simulink model "EOM"  (R2020a)
settings: Solver=VariableStepAuto  StartTime=0.0  StopTime=10.0  RelTol=1e-3
undefined symbols (not defined in the file): itki, Iyy, pos_ini, theta_ini, velbody_ini
libraries: simulink x1, aerolibatmos2 x1
settings Model: Creator=Emir  LastModifiedBy=benyo
settings DebuggingCC: UnconnectedInputMsg=none  UnconnectedOutputMsg=none  UnconnectedLineMsg=none  SFMachineParentedDataDiag=error

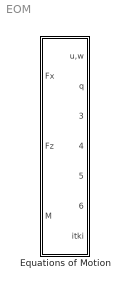
== system EOM ==
  Equations of Motion : Subsystem

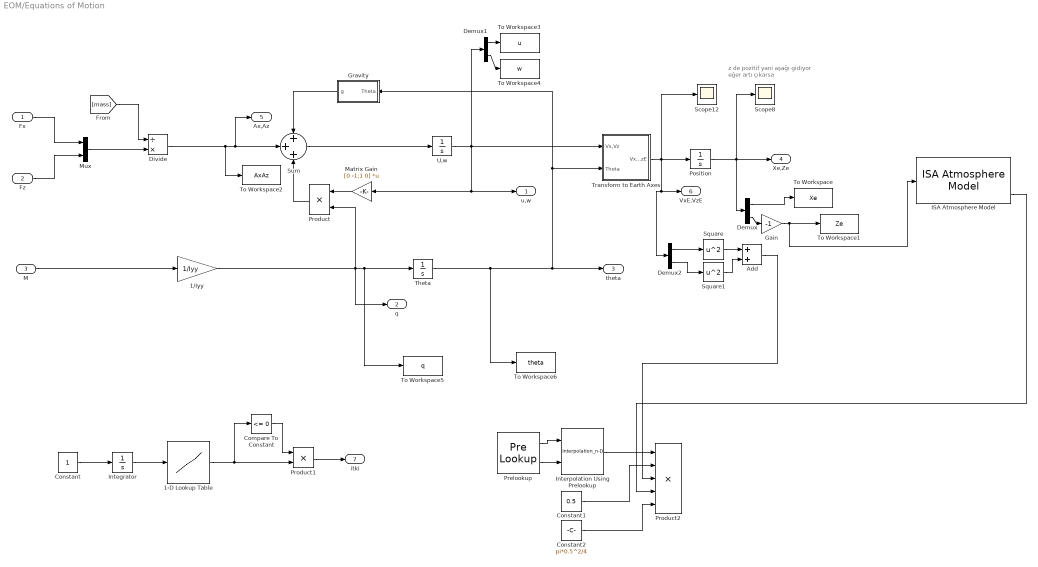
== system EOM/Equations of Motion ==
  note: z de pozitif yani aşağı
      | gidiyor eğer artı çıkarsa
  Fx : Inport
  Fz : Inport  Port=2
  M : Inport  Port=3
  1-D Lookup Table : Lookup_n-D  NumberOfTableDimensions=1  BreakpointsForDimension1=t  Table=itki  InternalRulePriority=Speed  RndMeth=Simplest  InputSameDT=on
  1/Iyy : Gain  Gain=1/Iyy  SaturateOnIntegerOverflow=on  OutDataTypeStr=Inherit: Same as input  ParamDataTypeStr=Inherit: Same as input
  Add : Sum
  Compare To Constant : simulink/Logic and Bit Operations/Compare To Constant  relop=<=  const=0  OutDataTypeStr=boolean
  Constant : Constant
  Constant1 : Constant  Value=0.5
  Constant2 : Constant  Value=pi*0.5^2/4
  Demux : Demux  Outputs=2
  Demux1 : Demux  Outputs=2
  Demux2 : Demux  Outputs=2
  Divide : Product  Inputs=/*
  Gain : Gain  Gain=-1
  Gravity : Subsystem
  ISA Atmosphere Model : aerolibatmos2/ISA Atmosphere Model  custom=off  g=9.80665  gamma=1.4  R=287.0531  L=0.0065  h_trop=11000  h_strat=20000  rho0=1.225  P0=101325  T0=288.15  h0=0
  Integrator : Integrator
  Interpolation Using Prelookup : Interpolation_n-D  NumberOfTableDimensions=1  InternalRulePriority=Speed
      settings: InputPortMap=u0,u1
  Matrix Gain : Gain  Gain=[0 -1;1 0]  Multiplication=Matrix(K*u)  SaturateOnIntegerOverflow=on  OutDataTypeStr=Inherit: Same as input  ParamDataTypeStr=Inherit: Same as input
  Mux : Mux  Inputs=2
  Position : Integrator  InitialCondition=pos_ini
  Prelookup : PreLookup  BreakpointsData=[10:10:110]  ExtrapMethod=Linear
  Product : Product  InputSameDT=on  RndMeth=Zero  SaturateOnIntegerOverflow=on  OutDataTypeStr=Inherit: Same as first input
  Product1 : Product
  Product2 : Product  Inputs=5
  Scope12 : Scope
  Scope8 : Scope
  Square : Math  Operator=square  SaturateOnIntegerOverflow=on
  Square1 : Math  Operator=square  SaturateOnIntegerOverflow=on
  Sum : Sum  Inputs=+++  InputSameDT=on  SaturateOnIntegerOverflow=on  OutDataTypeStr=Inherit: Same as first input
  Theta : Integrator  InitialCondition=theta_ini
  To Workspace : ToWorkspace  VariableName=Xe  SampleTime=-1
  To Workspace1 : ToWorkspace  VariableName=Ze  SampleTime=-1
  To Workspace2 : ToWorkspace  VariableName=AxAz  SaveFormat=Timeseries  SampleTime=-1
  To Workspace3 : ToWorkspace  VariableName=u  SaveFormat=Timeseries  SampleTime=-1
  To Workspace4 : ToWorkspace  VariableName=w  SaveFormat=Timeseries  SampleTime=-1
  To Workspace5 : ToWorkspace  VariableName=q  SampleTime=-1
  To Workspace6 : ToWorkspace  VariableName=theta  SampleTime=-1
  Transform to Earth Axes : Subsystem
  U,w : Integrator  InitialCondition=velbody_ini
  u,w : Outport
  q : Outport  Port=2
  theta : Outport  Port=3
  Xe,Ze : Outport  Port=4  InitialOutput=0
  Ax,Az : Outport  Port=5
  VxE,VzE : Outport  Port=6  InitialOutput=0
  itki : Outport  Port=7
  wires:
  Fx/1 -> Mux/1
  Fz/1 -> Mux/2
  Mux/1 -> Divide/2
  Divide/1 -> Sum/2, Ax,Az/1, To Workspace2/1
  Product/1 -> Sum/3
  Matrix Gain/1 -> Product/1
  1/Iyy/1 -> q/1, Theta/1, To Workspace5/1, Product/2
  Sum/1 -> U,w/1
  Theta/1 -> theta/1, Gravity/1(Theta), Transform to Earth Axes/2(Theta), To Workspace6/1
  Gravity/1(g) -> Sum/1
  U,w/1 -> Transform to Earth Axes/1(Vx,Vz), Matrix Gain/1, u,w/1, Demux1/1
  M/1 -> 1/Iyy/1
  Position/1 -> Scope8/1, Xe,Ze/1, Demux/1
  Transform to Earth Axes/1(VxE,VzE) -> Position/1, Scope12/1, VxE,VzE/1, Demux2/1
  [mass] -> Divide/1
  Demux/1 -> To Workspace/1
  Demux/2 -> Gain/1
  Gain/1 -> To Workspace1/1, ISA Atmosphere Model/1
  Demux1/1 -> To Workspace3/1
  Demux1/2 -> To Workspace4/1
  Constant/1 -> Integrator/1
  Integrator/1 -> 1-D Lookup Table/1
  1-D Lookup Table/1 -> Compare To Constant/1, Product1/2
  Compare To Constant/1 -> Product1/1
  Product1/1 -> itki/1
  Prelookup/1 -> Interpolation Using Prelookup/1
  Prelookup/2 -> Interpolation Using Prelookup/2
  Interpolation Using Prelookup/1 -> Product2/1
  Constant1/1 -> Product2/2
  Demux2/1 -> Square/1
  Demux2/2 -> Square1/1
  Square/1 -> Add/1
  Square1/1 -> Add/2
  Add/1 -> Product2/3
  ISA Atmosphere Model/4 -> Product2/4
  Constant2/1 -> Product2/5

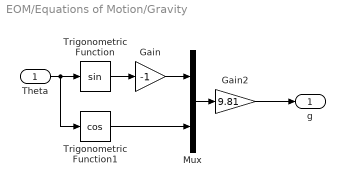
== system EOM/Equations of Motion/Gravity ==
  Theta : Inport
  Gain : Gain  Gain=-1  SaturateOnIntegerOverflow=on  OutDataTypeStr=Inherit: Same as input  ParamDataTypeStr=Inherit: Same as input
  Gain2 : Gain  Gain=9.81  SaturateOnIntegerOverflow=on  OutDataTypeStr=Inherit: Same as input  ParamDataTypeStr=Inherit: Same as input
  Mux : Mux  Inputs=2
  Trigonometric Function : Trigonometry
  Trigonometric Function1 : Trigonometry  Operator=cos
  g : Outport
  wires:
  Gain2/1 -> g/1
  Mux/1 -> Gain2/1
  Trigonometric Function1/1 -> Mux/2
  Gain/1 -> Mux/1
  Trigonometric Function/1 -> Gain/1
  Theta/1 -> Trigonometric Function/1, Trigonometric Function1/1

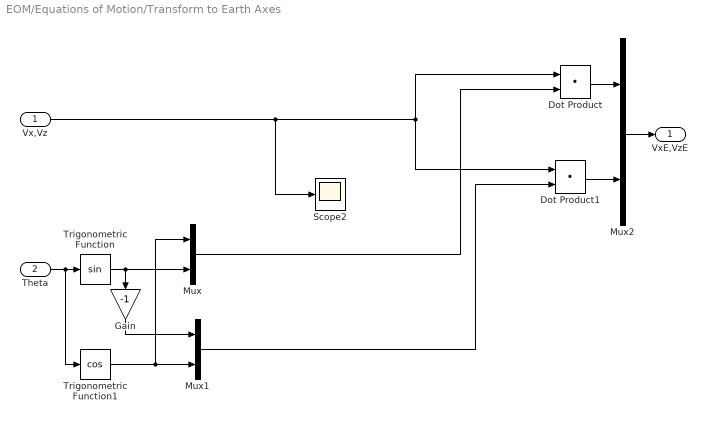
== system EOM/Equations of Motion/Transform to Earth Axes ==
  Vx,Vz : Inport
  Theta : Inport  Port=2
  Dot Product : DotProduct  InputSameDT=on  OutDataTypeStr=Inherit: Inherit via internal rule
  Dot Product1 : DotProduct  InputSameDT=on  OutDataTypeStr=Inherit: Inherit via internal rule
  Gain : Gain  Gain=-1  SaturateOnIntegerOverflow=on  OutDataTypeStr=Inherit: Same as input  ParamDataTypeStr=Inherit: Same as input
  Mux : Mux  Inputs=2
  Mux1 : Mux  Inputs=2
  Mux2 : Mux  Inputs=2
  Scope2 : Scope
  Trigonometric Function : Trigonometry
  Trigonometric Function1 : Trigonometry  Operator=cos
  VxE,VzE : Outport
  wires:
  Gain/1 -> Mux1/1
  Trigonometric Function/1 -> Mux/2, Gain/1
  Theta/1 -> Trigonometric Function1/1, Trigonometric Function/1
  Mux/1 -> Dot Product/2
  Mux2/1 -> VxE,VzE/1
  Dot Product1/1 -> Mux2/2
  Dot Product/1 -> Mux2/1
  Mux1/1 -> Dot Product1/2
  Trigonometric Function1/1 -> Mux1/2, Mux/1
  Vx,Vz/1 -> Dot Product/1, Dot Product1/1, Scope2/1
